simulink model "Animation_Simulink"  (R2020a)
settings: Solver=FixedStepDiscrete  StartTime=0.0  StopTime=max(t)-1/FR  FixedStep=1/FR  RelTol=1e-3
values from neighbouring files (symbols this model uses):
  FR = Bodies.System.FR    [S_Function_Animation.m]    (also in fft_study.m; plot_relative_data.m)
libraries: vrlib x1
settings Model: Creator=1511 IRON  LastModifiedBy=1511 IRON
settings DataIOCC: ExternalInput=d_Ang_ord

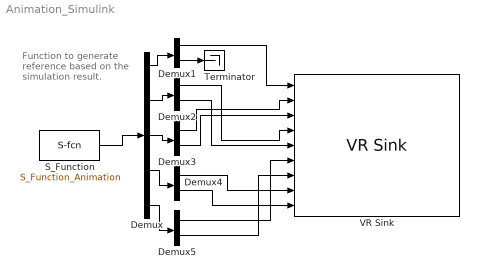
== system Animation_Simulink ==
  note: Function to generate reference based on the simulation result.
  Demux : Demux  Outputs=5
  Demux{1..5} (5 alike) : Demux  Outputs=2
  S_Function : S-Function  FunctionName=S_Function_Animation  SFunctionDeploymentMode=off  EnableBusSupport=off
  Terminator : Terminator
  VR Sink : vrlib/VR Sink  InstantiateOnLoad=on  SampleTime=1/FR  ViewEnable=on  RemoteChange=off  RemoteView=off  FieldsWritten=HUB.rotation.4.1.1.double#SIP.rotation.4.1.1.double#SIP.translation.3.1.1.double#SLP.rotation.4.1.1.double#SLP.translation.3.1.1.double#E_Field_Pos.rotation.4.1.1.double#E_Field_Pos.translation.3.1.1.double#E_Field_Neg.rotation.4.1.1.double#E_Field_Neg.translation.3.1.1.double  WorldFileName=Modelo_3D.x3d  AutoView=on  VideoDimensions=[]  AllowVariableSize=off  FigureProperties="{'Position', 'Name', 'Viewpoint', 'CameraBound', 'CameraDirection', 'CameraPosition', 'CameraUpVector', 'ZoomFactor', 'Antialiasing', 'Headlight', 'Lighting', 'NavPanel', 'Sound', 'StatusBar', 'Stereo3D', 'Stereo3DCameraOffset', 'Stereo3DHIT', 'ToolBar', 'Textures', 'Transparency', 'Triad', 'Wireframe', 'NavZones', 'NavMode', 'NavSpeed', 'CaptureFileFormat', 'CaptureFileName', 'Record2DCompressMethod', 'Record2DCompressQuality', 'Record2D', 'Record2DFileName', 'Record2DFPS'; [7.9000000000000000e+02   4.0900000000000000e+02   9.5800000000000000e+02   3.8400000000000000e+02], '', '', 'on', [4.0089261391941472e-01   2.3722834861727174e-01  -8.8487729246331159e-01], [-1.0586188017167026e+00  -1.6788205673369155e-01   1.1946847206464570e+00], [4.9926654326721068e-02   9.5879856024342103e-01   2.7966524643383267e-01], [1.0000000000000000e+00], 'on', 'on', 'on', 'halfbar', 'on', 'on', 'off', [1.0000000149011612e-01], [0.0000000000000000e+00], 'on', 'on', 'on', 'bottomleft', 'off', 'off', 'examine', 'normal', 'tif', '%f_anim_%n.tif', 'auto', [1.0000000000000000e+02], 'off', '%f_anim_%n.avi', 'auto'}"
  wires:
  S_Function/1 -> Demux/1
  Demux/1 -> Demux1/1
  Demux/2 -> Demux2/1
  Demux/3 -> Demux3/1
  Demux/4 -> Demux4/1
  Demux/5 -> Demux5/1
  Demux1/1 -> VR Sink/1
  Demux3/1 -> VR Sink/2
  Demux2/1 -> VR Sink/4
  Demux5/1 -> VR Sink/6
  Demux4/1 -> VR Sink/8
  Demux3/2 -> VR Sink/3
  Demux4/2 -> VR Sink/9
  Demux5/2 -> VR Sink/7
  Demux2/2 -> VR Sink/5
  Demux1/2 -> Terminator/1
